simulink model "punto7"  (R2015a)
settings: Solver=ode45  StartTime=0.0  StopTime=10.0  RelTol=1e-3
libraries: simulink x2
settings Model: Creator=Administrador  LastModifiedBy=Administrador

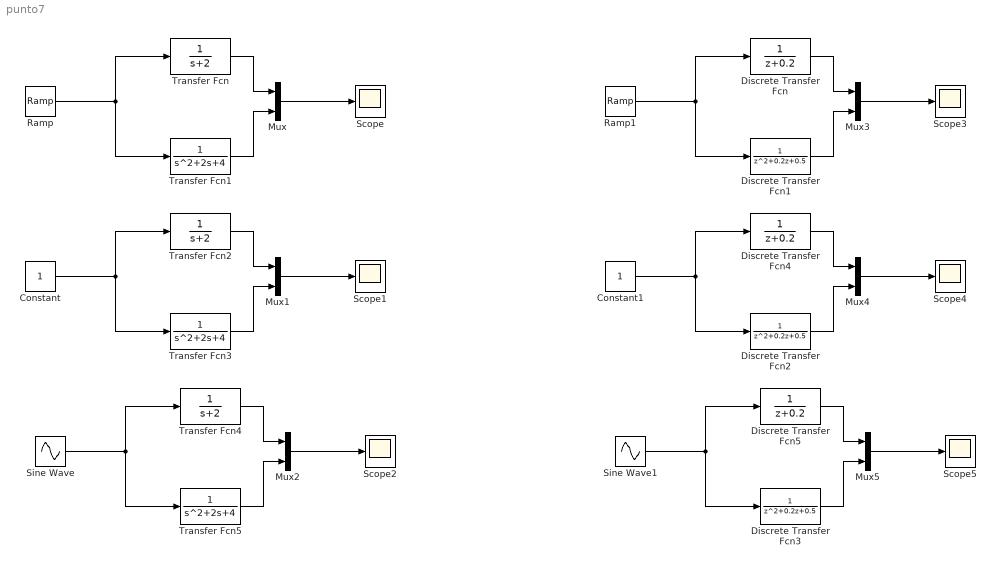
== system punto7 ==
  Constant : Constant
  Constant1 : Constant
  Discrete Transfer Fcn : DiscreteTransferFcn  Denominator=[1 0.2]  SampleTime=0.1
  Discrete Transfer Fcn1 : DiscreteTransferFcn  Denominator=[1 0.2 0.5]  SampleTime=0.1
  Discrete Transfer Fcn2 : DiscreteTransferFcn  Denominator=[1 0.2 0.5]  SampleTime=0.1
  Discrete Transfer Fcn3 : DiscreteTransferFcn  Denominator=[1 0.2 0.5]  SampleTime=0.1
  Discrete Transfer Fcn4 : DiscreteTransferFcn  Denominator=[1 0.2]  SampleTime=0.1
  Discrete Transfer Fcn5 : DiscreteTransferFcn  Denominator=[1 0.2]  SampleTime=0.1
  Mux{,1..5} (6 alike) : Mux  Inputs=2
  Ramp : simulink/Sources/Ramp  slope=1  start=0  X0=1
  Ramp1 : simulink/Sources/Ramp  slope=1  start=0  X0=1
  Scope{,1..5} (6 alike) : Scope
      Scope2 settings: SaveName=ScopeData2
      Scope3 settings: SaveName=ScopeData3
      Scope4 settings: SaveName=ScopeData4
      Scope5 settings: SaveName=ScopeData5
  Sine Wave : Sin  SampleTime=0
  Sine Wave1 : Sin  SampleTime=0
  Transfer Fcn : TransferFcn  Denominator=[1 2]
  Transfer Fcn1 : TransferFcn  Denominator=[1 2 4]
  Transfer Fcn2 : TransferFcn  Denominator=[1 2]
  Transfer Fcn3 : TransferFcn  Denominator=[1 2 4]
  Transfer Fcn4 : TransferFcn  Denominator=[1 2]
  Transfer Fcn5 : TransferFcn  Denominator=[1 2 4]
  wires:
  Mux/1 -> Scope/1
  Transfer Fcn/1 -> Mux/1
  Transfer Fcn1/1 -> Mux/2
  Ramp/1 -> Transfer Fcn1/1, Transfer Fcn/1
  Mux1/1 -> Scope1/1
  Transfer Fcn2/1 -> Mux1/1
  Transfer Fcn3/1 -> Mux1/2
  Constant/1 -> Transfer Fcn3/1, Transfer Fcn2/1
  Mux2/1 -> Scope2/1
  Transfer Fcn4/1 -> Mux2/1
  Transfer Fcn5/1 -> Mux2/2
  Sine Wave/1 -> Transfer Fcn5/1, Transfer Fcn4/1
  Mux3/1 -> Scope3/1
  Discrete Transfer Fcn/1 -> Mux3/1
  Discrete Transfer Fcn1/1 -> Mux3/2
  Ramp1/1 -> Discrete Transfer Fcn1/1, Discrete Transfer Fcn/1
  Mux4/1 -> Scope4/1
  Discrete Transfer Fcn4/1 -> Mux4/1
  Discrete Transfer Fcn2/1 -> Mux4/2
  Constant1/1 -> Discrete Transfer Fcn4/1, Discrete Transfer Fcn2/1
  Mux5/1 -> Scope5/1
  Discrete Transfer Fcn5/1 -> Mux5/1
  Discrete Transfer Fcn3/1 -> Mux5/2
  Sine Wave1/1 -> Discrete Transfer Fcn5/1, Discrete Transfer Fcn3/1
